simulink subsystem "Ultrasonidos"  (R2022b)
settings: Solver=VariableStepAuto  StartTime=0.0  StopTime=10.0  RelTol=1e-3
libraries: arduinolib x2
settings Model: Creator=Usuario_UMA  LastModifiedBy=Usuario
settings OptimizationCC: ReuseModelBlockBuffer=on

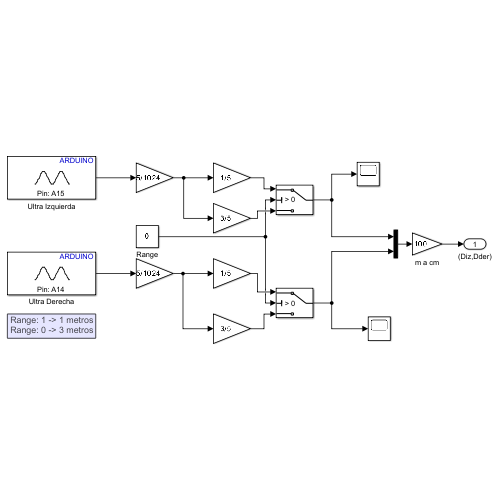
[thumbnail: Simulink's stored preview of the top-level diagram]
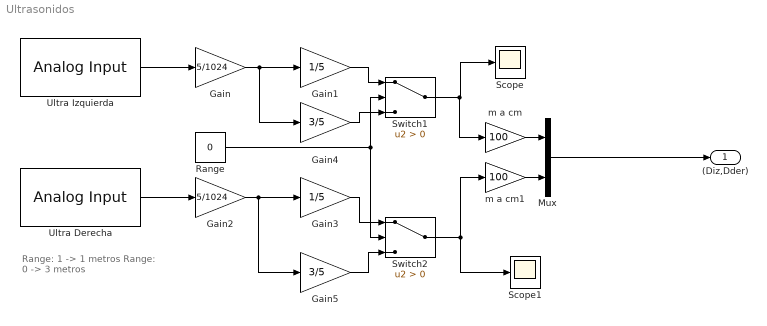
== system Ultrasonidos ==
  note: Range: 1 -> 1 metros
      | Range: 0 -> 3 metros
  Gain : Gain  Gain=5/1024  OutDataTypeStr=double
  Gain1 : Gain  Gain=1/5
  Gain2 : Gain  Gain=5/1024  OutDataTypeStr=double
  Gain3 : Gain  Gain=1/5
  Gain4 : Gain  Gain=3/5
  Gain5 : Gain  Gain=3/5
  Mux : Mux  Inputs=2
  Range : Constant  Value=0
  Scope : Scope
  Scope1 : Scope
  Switch1 : Switch  Criteria=u2 > Threshold  SaturateOnIntegerOverflow=off  InputSameDT=off
  Switch2 : Switch  Criteria=u2 > Threshold  SaturateOnIntegerOverflow=off  InputSameDT=off
  Ultra Derecha : arduinolib/Analog Input  pinNumber=14  ReadResultsOnly=off  ConversionTriggerSource=Software  ExternalTriggerType=uint32( 0 )  OutputDataType=uint16  EnableConversionCompleteNotify=off  EnableOuputStatus=off  SampleTime=-1  blockPlatform=arduino
  Ultra Izquierda : arduinolib/Analog Input  pinNumber=15  ReadResultsOnly=off  ConversionTriggerSource=Software  ExternalTriggerType=uint32( 0 )  OutputDataType=uint16  EnableConversionCompleteNotify=off  EnableOuputStatus=off  SampleTime=-1  blockPlatform=arduino
  m a cm : Gain  Gain=100
  m a cm1 : Gain  Gain=100
  (Diz,Dder) : Outport
  wires:
  m a cm1/1 -> Mux/2
  m a cm/1 -> Mux/1
  Mux/1 -> (Diz,Dder)/1
  Range/1 -> Switch2/2, Switch1/2
  Gain1/1 -> Switch1/1
  Switch1/1 -> m a cm/1, Scope/1
  Ultra Izquierda/1 -> Gain/1
  Switch2/1 -> m a cm1/1, Scope1/1
  Gain5/1 -> Switch2/3
  Gain3/1 -> Switch2/1
  Gain4/1 -> Switch1/3
  Gain2/1 -> Gain3/1, Gain5/1
  Ultra Derecha/1 -> Gain2/1
  Gain/1 -> Gain1/1, Gain4/1
